simulink model "BatteryModel_Solution"  (R2025a)
settings: Solver=VariableStepAuto  StartTime=0.0  StopTime=3600  RelTol=1e-3
undefined symbols (not defined in the file): Cn, I, OCV, R_Charge, R_Discharge, SOC
settings Model: Creator=Pablo  LastModifiedBy=Pablo

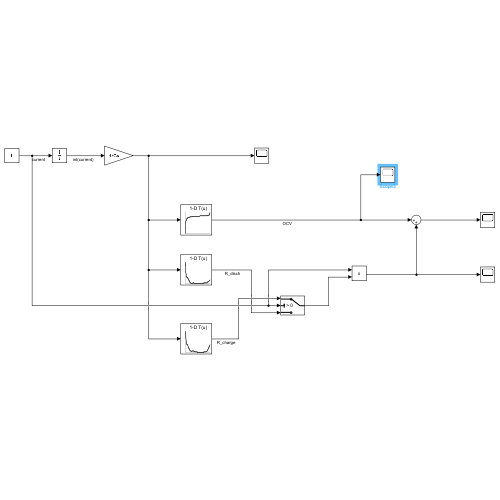
[thumbnail: Simulink's stored preview of the top-level diagram]
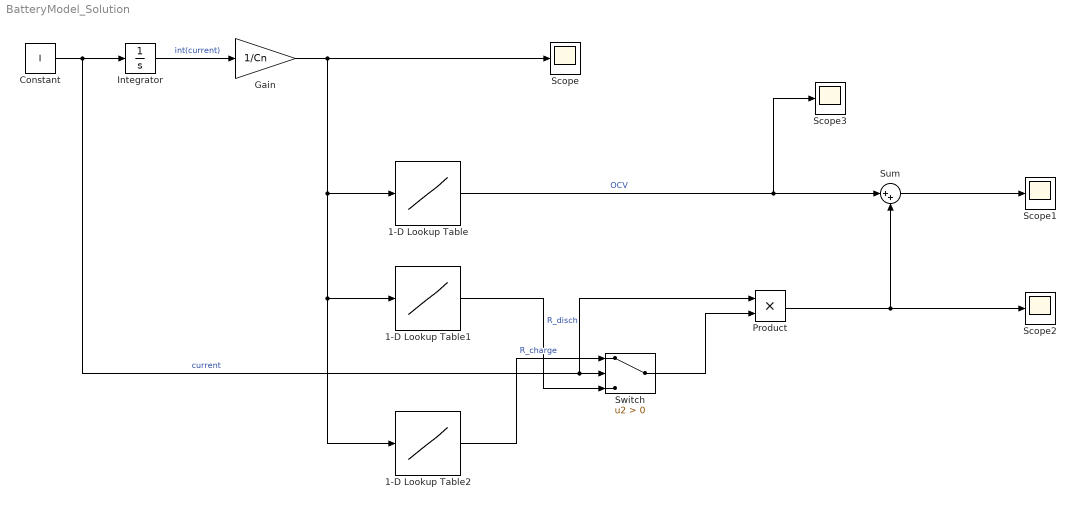
== system BatteryModel_Solution ==
  1-D Lookup Table : Lookup_n-D  NumberOfTableDimensions=1  BreakpointsForDimension1=SOC  Table=OCV  InternalRulePriority=Speed  RndMeth=Simplest
  1-D Lookup Table1 : Lookup_n-D  NumberOfTableDimensions=1  BreakpointsForDimension1=SOC  Table=R_Discharge  InternalRulePriority=Speed  RndMeth=Simplest
  1-D Lookup Table2 : Lookup_n-D  NumberOfTableDimensions=1  BreakpointsForDimension1=SOC  Table=R_Charge  InternalRulePriority=Speed  RndMeth=Simplest
  Constant : Constant  Value=I
  Gain : Gain  Gain=1/Cn
  Integrator : Integrator
  Product : Product
  Scope{,1..3} (4 alike) : Scope
      Scope1 settings: ActiveDisplayYMinimum=2.5431799999999987  ActiveDisplayYMaximum=4.7913800000000135
      Scope2 settings: ActiveDisplayYMinimum=0.15657628926513256  ActiveDisplayYMaximum=0.39149152341498533  DataLoggingVariableName=ScopeData2
      Scope3 settings: ActiveDisplayYMinimum=2.1599999999999984  ActiveDisplayYMaximum=4.5600000000000138  DataLoggingVariableName=ScopeData3
  Sum : Sum  Inputs=|++
  Switch : Switch  Criteria=u2 > Threshold  SaturateOnIntegerOverflow=off  InputSameDT=off
  wires:
  Constant/1 -> Product/1, Switch/2, Integrator/1  "current"
  Integrator/1 -> Gain/1  "int(current)"
  Gain/1 -> 1-D Lookup Table/1, 1-D Lookup Table2/1, 1-D Lookup Table1/1, Scope/1
  1-D Lookup Table2/1 -> Switch/1  "R_charge"
  1-D Lookup Table1/1 -> Switch/3  "R_disch"
  1-D Lookup Table/1 -> Scope3/1, Sum/1  "OCV"
  Switch/1 -> Product/2
  Product/1 -> Scope2/1, Sum/2
  Sum/1 -> Scope1/1
